simulink model "untitled"  (R2022b)
settings: Solver=VariableStepAuto  StartTime=0.0  StopTime=5  RelTol=1e-3
settings Model: Creator=24424  LastModifiedBy=24424

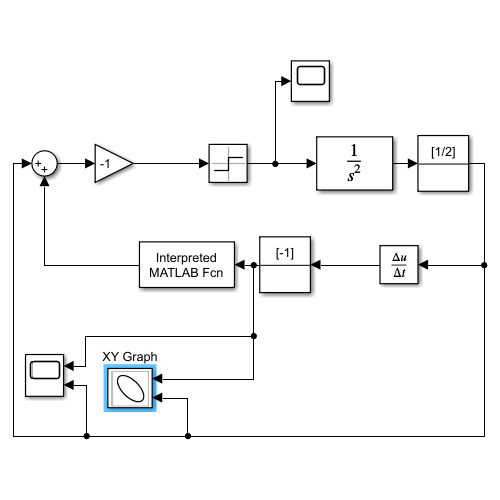
[thumbnail: Simulink's stored preview of the top-level diagram]
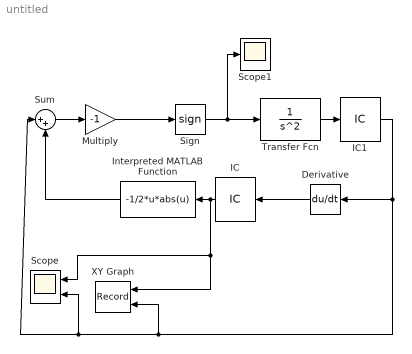
== system untitled ==
  Derivative : Derivative
  IC : InitialCondition  Value=-1
  IC1 : InitialCondition  Value=1/2
  Interpreted MATLAB Function : MATLABFcn  MATLABFcn=-1/2*u*abs(u)
  Multiply : Gain  Gain=-1
  Scope : Scope  NumInputPorts=2
  Scope1 : Scope
  Sign : Signum  ZeroCross=off
  Sum : Sum  Inputs=|++
  Transfer Fcn : TransferFcn  Denominator=[1 0 0]
  XY Graph : Record  FileSettingsInternal="{\"entries\":[{\"content\":{\"excelSettings\":{\"content\":{},\"type\":\"Streamout.ExcelSettings\"}},\"type\":\"Streamout.FileSettingStorage\",\"uuid\":\"cef5a93a-f6c0-4737-9fe1-225a539e6c7b\"}],\"packageUris\":[\"http://schema.mathworks.com/mf0/streamout_blocks/R2020a\"],\"version\":\"1.0\"}"  Layout=[1 1]  SignalsInternal="{\"entries\":[{\"content\":{\"signals\":[{\"content\":{\"blockPath\":[\"untitled/XY Graph\"],\"channel\":[],\"dimensions\":[1],\"domain\":\"untitled/XY Graph\",\"lineColor\":\"#a2142f\",\"plots\":[1],\"port\":1,\"sid\":[\"\"],\"signalID\":5560,\"signalName\":\"IC\"},\"type\":\"RecordBlkView.Signal\",\"uuid\":\"f0def155-1e52-44e3-aee1-00a9d3aa7648\"},{\"content\":{\"blockPath\":[\"untitled/XY Graph\"],\"channel\":[],\"dimensions\":[1],\"domain\":\"untitled/XY Graph\",\"lineColor\":\"#139fff\",\"plots\":[1],\"port\":2,\"sid\":[\"\"],\"signalID\":5564,\"signalName\":\"IC1\"},\"type\":\"RecordBlkView.Signal\",\"uuid\":\"1927c63d-cb56-4f0e-bf62-336fc04be01c\"}]},\"type\":\"RecordBlkView.InputSignals\",\"uuid\":\"b1f5d4f7-4381-4aa8-be12-db12744cb678\"}],\"packageUris\":[\"http://schema.mathworks.com/mf0/streamout_blocks/R2020a\"],\"version\":\"1.0\"}"  VisualizationBindings="{\"xyplotplugin\":{\"info\":[{\"series\":[{\"bindingParametersList\":[{\"parameter\":\"X-Axis\",\"signalID\":5560,\"signalName\":\"IC\"},{\"parameter\":\"Y-Axis\",\"signalID\":5564,\"signalName\":\"IC1\"}],\"seriesID\":42949}],\"subplotID\":1}]}}"  CompatibilityTag=XY
  wires:
  Sum/1 -> Multiply/1
  Multiply/1 -> Sign/1
  Sign/1 -> Scope1/1, Transfer Fcn/1
  Transfer Fcn/1 -> IC1/1
  Interpreted MATLAB Function/1 -> Sum/2
  IC1/1 -> XY Graph/2, Scope/2, Sum/1, Derivative/1
  Derivative/1 -> IC/1
  IC/1 -> Scope/1, XY Graph/1, Interpreted MATLAB Function/1
